simulink model "Simulator"  (R2020a)
settings: Solver=VariableStepAuto  StartTime=0.0  StopTime=100  RelTol=1e-3
libraries: robotmobilelib x1
settings Model: Creator=vinic  LastModifiedBy=vinic

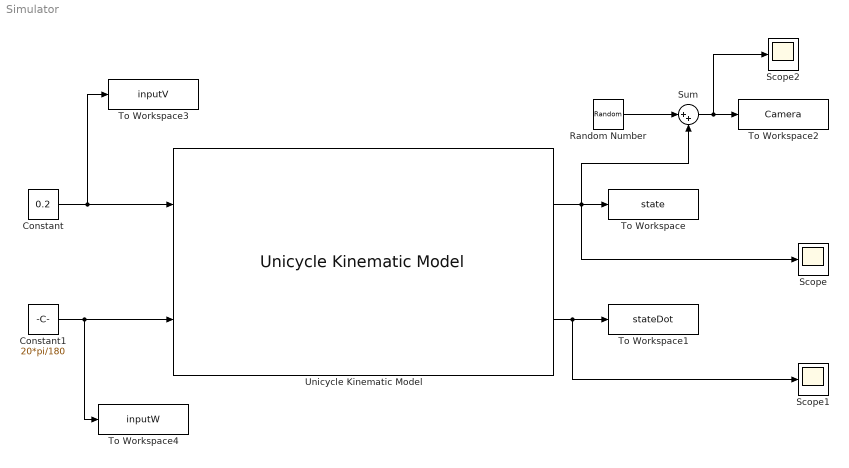
== system Simulator ==
  Constant : Constant  Value=0.2  SampleTime=1/30
  Constant1 : Constant  Value=20*pi/180  SampleTime=1/30
  Random Number : RandomNumber  Variance=0.005  SampleTime=1/30
  Scope : Scope
  Scope1 : Scope
  Scope2 : Scope
  Sum : Sum  Inputs=|++
  To Workspace : ToWorkspace  VariableName=state  SaveFormat=Timeseries  SampleTime=-1
  To Workspace1 : ToWorkspace  VariableName=stateDot  SaveFormat=Timeseries  SampleTime=-1
  To Workspace2 : ToWorkspace  VariableName=Camera  SaveFormat=Timeseries  SampleTime=-1
  To Workspace3 : ToWorkspace  VariableName=inputV  SaveFormat=Timeseries  SampleTime=-1
  To Workspace4 : ToWorkspace  VariableName=inputW  SaveFormat=Timeseries  SampleTime=-1
  Unicycle Kinematic Model : robotmobilelib/Unicycle Kinematic Model  VehicleInputs=Vehicle Speed & Heading Angular Velocity  WheelRadius=0.1  WheelSpeedRange=[-2 2]  InitialState=[0; 0; 0]  SimulateUsing=Interpreted execution
      settings: SourceProductBaseCode=RO
  wires:
  Constant/1 -> To Workspace3/1, Unicycle Kinematic Model/1
  Constant1/1 -> To Workspace4/1, Unicycle Kinematic Model/2
  Unicycle Kinematic Model/1 -> Sum/2, To Workspace/1, Scope/1
  Unicycle Kinematic Model/2 -> Scope1/1, To Workspace1/1
  Random Number/1 -> Sum/1
  Sum/1 -> Scope2/1, To Workspace2/1
